simulink subsystem "InversePendulum"  (R2023a)
settings: Solver=VariableStepAuto  StartTime=0.0  StopTime=10.0  RelTol=1e-3
undefined symbols (not defined in the file): ProjectPend
settings Model: Creator=Лиза  LastModifiedBy=mrrom

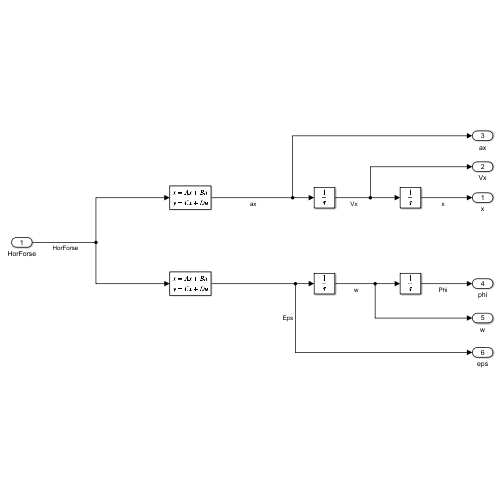
[thumbnail: Simulink's stored preview of the top-level diagram]
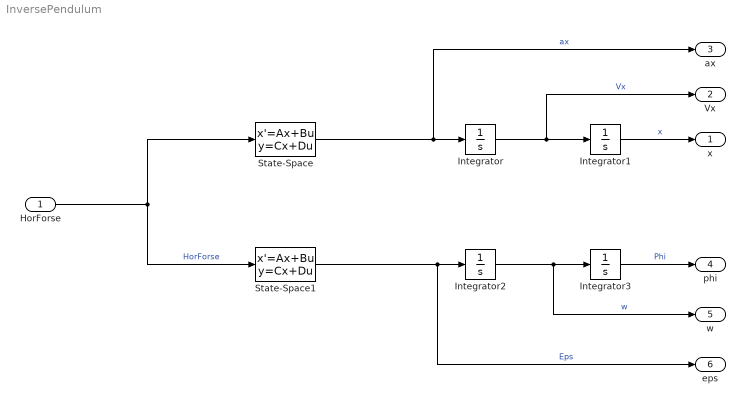
== system InversePendulum ==
  HorForse : Inport
  Integrator{,1..3} (4 alike) : Integrator
  State-Space : StateSpace  A=ProjectPend.A  B=ProjectPend.B  C="[ 0      0          (ProjectPend.m^2*ProjectPend.g*ProjectPend.l^2)/ProjectPend.p   0]"  D=[(ProjectPend.I+ProjectPend.m*ProjectPend.l^2)/ProjectPend.p]  InitialCondition=ProjectPend.Init_St
  State-Space1 : StateSpace  A=ProjectPend.A  B=ProjectPend.B  C=[ 0 0 -ProjectPend.m*ProjectPend.g*ProjectPend.l*(ProjectPend.M+ProjectPend.m)/ProjectPend.p 0]  D=-ProjectPend.m*ProjectPend.l/ProjectPend.p  InitialCondition=ProjectPend.Init_St
  x : Outport
  Vx : Outport  Port=2
  ax : Outport  Port=3
  phi : Outport  Port=4
  w : Outport  Port=5
  eps : Outport  Port=6
  wires:
  HorForse/1 -> State-Space1/1, State-Space/1  "HorForse"
  State-Space/1 -> ax/1, Integrator/1  "ax"
  Integrator/1 -> Vx/1, Integrator1/1  "Vx"
  State-Space1/1 -> eps/1, Integrator2/1  "Eps"
  Integrator2/1 -> w/1, Integrator3/1  "w"
  Integrator1/1 -> x/1  "x"
  Integrator3/1 -> phi/1  "Phi"
